simulink model "LQG_tracker_discrete_time"  (R2025b)
settings: Solver=VariableStepAuto  StartTime=0.0  StopTime=10.0  FixedStep=Ts  RelTol=1e-3
values from neighbouring files (symbols this model uses):
  A = [ 0, 1, 0, 0 ... (first row only)    [Controller_LQR.m]    (also in H_inf_controller.m = zeros(4,4); Hinf.m = zeros(4,4); Hinf_tuner.m = zeros(4,4); LQG_controller.m = zeros(4,4))
  B = [0 ... (first row only)    [Controller_LQR.m]    (also in H_inf_controller.m = (dx_p - dx_m) / (2*h); Hinf.m = (dx_p - dx_m) / (2*h); Hinf_tuner.m = (dx_p - dx_m)/(2*h); LQG_controller.m = (dx_p - dx_m) / (2*h))
  C = [1 0 0 0]    [Controller_LQR.m]    (also in H_inf_controller.m; Hinf.m; Hinf_tuner.m; LQG_controller.m)
  D = 0    [Controller_LQR.m]    (also in H_inf_controller.m; Hinf.m; Hinf_tuner.m; LQG_controller.m)
  sys_plant_d = c2d(sys_plant, Ts, 'zoh')    [LQG_controller.m]
  Ts = 0.01    [Hinf.m]    (also in Hinf_tuner.m; LQG_controller.m; MPC_controller.m; helicopter_lqg_design.m)
settings Model: Creator=Administrator  LastModifiedBy=Administrator

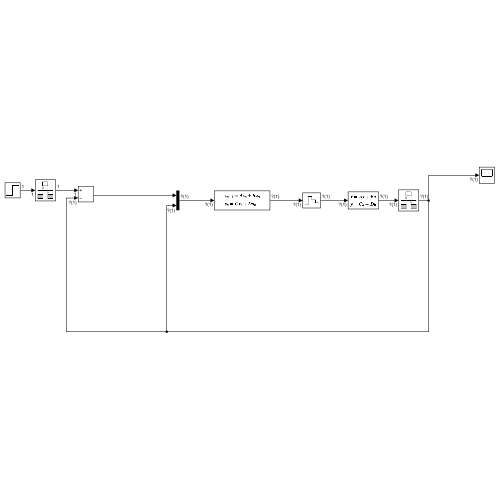
[thumbnail: Simulink's stored preview of the top-level diagram]
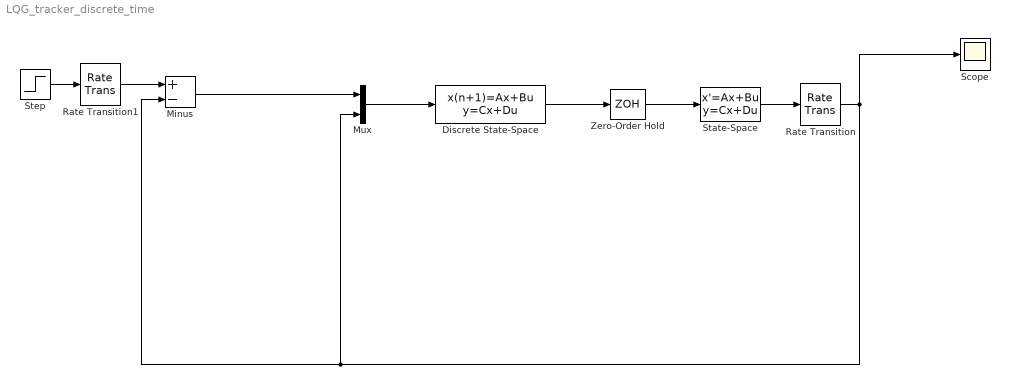
== system LQG_tracker_discrete_time ==
  Discrete State-Space : DiscreteStateSpace  A=sys_plant_d.A  B=sys_plant_d.B  C=sys_plant_d.C  D=sys_plant_d.D  SampleTime=Ts
  Minus : Sum  Inputs=+-
  Mux : Mux  Inputs=2
  Rate Transition : RateTransition  OutPortSampleTime=Ts
  Rate Transition1 : RateTransition  OutPortSampleTime=Ts
  Scope : Scope
      settings: ActiveDisplayYMinimum=-0.1264885247503322  ActiveDisplayYMaximum=1.13839672275299
  State-Space : StateSpace  A=A  B=B  C=C  D=D  InitialCondition=0
  Step : Step  SampleTime=0
  Zero-Order Hold : ZeroOrderHold  SampleTime=Ts
  wires:
  Discrete State-Space/1 -> Zero-Order Hold/1
  Zero-Order Hold/1 -> State-Space/1
  Mux/1 -> Discrete State-Space/1
  Minus/1 -> Mux/1
  State-Space/1 -> Rate Transition/1
  Rate Transition/1 -> Mux/2, Minus/2, Scope/1
  Step/1 -> Rate Transition1/1
  Rate Transition1/1 -> Minus/1
